simulink model "lista1_questao6_comparacao"  (R2014b)
settings: Solver=ode45  StartTime=0.0  StopTime=60  RelTol=1e-3
libraries: cstblocks x3
settings Model: Creator=Danilo  LastModifiedBy=Danilo

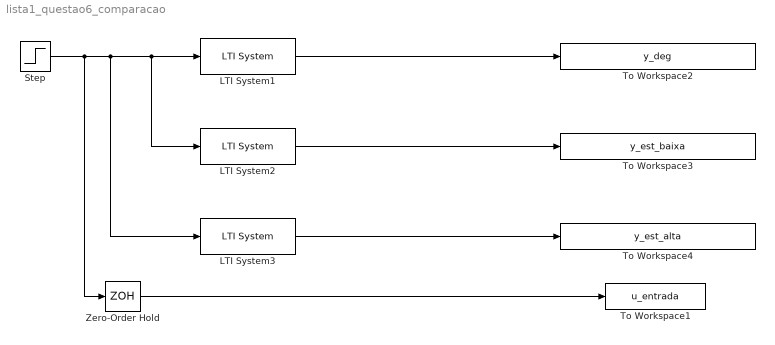
== system lista1_questao6_comparacao ==
  LTI System1 : cstblocks/LTI System  sys=H  IC=[]
  LTI System2 : cstblocks/LTI System  sys=H_est_baixa  IC=[]
  LTI System3 : cstblocks/LTI System  sys=H_est_alta  IC=[]
  Step : Step  SampleTime=1
  To Workspace1 : ToWorkspace  VariableName=u_entrada  SampleTime=1
  To Workspace2 : ToWorkspace  VariableName=y_deg  SampleTime=1
  To Workspace3 : ToWorkspace  VariableName=y_est_baixa  SampleTime=1
  To Workspace4 : ToWorkspace  VariableName=y_est_alta  SampleTime=1
  Zero-Order Hold : ZeroOrderHold
  wires:
  LTI System1/1 -> To Workspace2/1
  Step/1 -> Zero-Order Hold/1, LTI System3/1, LTI System2/1, LTI System1/1
  Zero-Order Hold/1 -> To Workspace1/1
  LTI System2/1 -> To Workspace3/1
  LTI System3/1 -> To Workspace4/1
